simulink library "Springs_Axle3_Independent"  (R2026a)
settings: Solver=VariableStepAuto
libraries: fl_lib x6, Spring_Element x6
Description:
  | Component of Simscape Vehicle Templates Library
  | 
  | Copyright 2018-2026 The MathWorks, Inc.
settings Model: Creator=smiller  LastModifiedBy=smiller

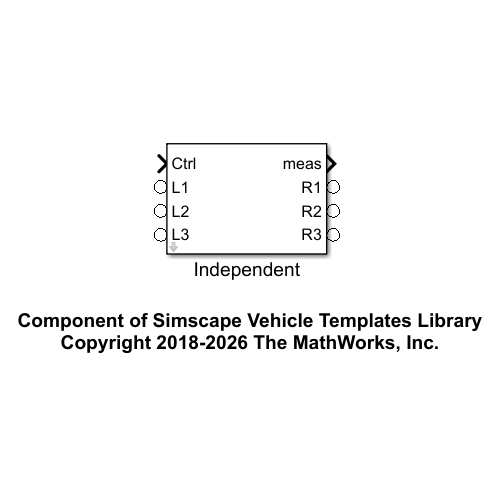
[thumbnail: Simulink's stored preview of the top-level diagram]
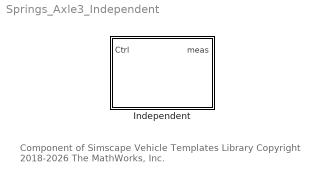
== system Springs_Axle3_Independent ==
  note: Component of Simscape Vehicle Templates Library
      | Copyright 2018-2026 The MathWorks, Inc.
  Independent : Subsystem  VariantControl=Independent  mask(Independent Springs){}
      mask help: Models independent left and right springs on three axles

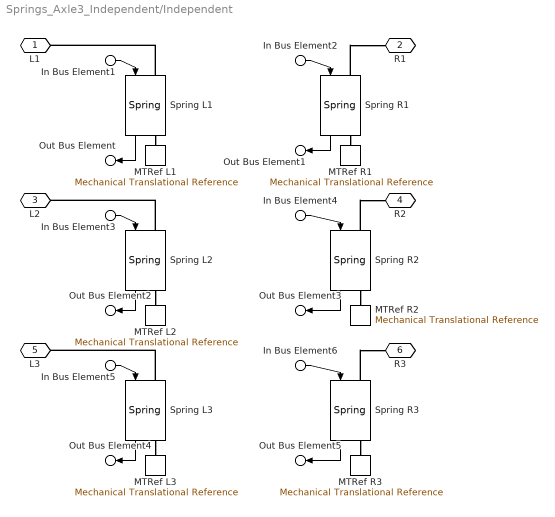
== system Springs_Axle3_Independent/Independent ==
  In Bus Element1 : Inport  PortName=Ctrl  Element=L1
  In Bus Element2 : Inport  PortName=Ctrl  Element=R1
  In Bus Element3 : Inport  PortName=Ctrl  Element=L2
  In Bus Element4 : Inport  PortName=Ctrl  Element=R2
  In Bus Element5 : Inport  PortName=Ctrl  Element=L3
  In Bus Element6 : Inport  PortName=Ctrl  Element=R3
  MTRef L1 : fl_lib/Mechanical/Translational Elements/Mechanical Translational Reference
  MTRef L2 : fl_lib/Mechanical/Translational Elements/Mechanical Translational Reference
  MTRef L3 : fl_lib/Mechanical/Translational Elements/Mechanical Translational Reference
  MTRef R1 : fl_lib/Mechanical/Translational Elements/Mechanical Translational Reference
  MTRef R2 : fl_lib/Mechanical/Translational Elements/Mechanical Translational Reference
  MTRef R3 : fl_lib/Mechanical/Translational Elements/Mechanical Translational Reference
  Spring L1 : Spring_Element/Spring  VariantControl=Variant1  LabelModeActiveChoice=Linear  Spring=Spring.Axle1  VariantLabel=Spring.Axle1.class.Value
      settings: AttributesFormatString=%<ActiveVariant>
  Spring L2 : Spring_Element/Spring  VariantControl=Variant1  LabelModeActiveChoice=Linear  Spring=Spring.Axle2  VariantLabel=Spring.Axle2.class.Value
      settings: AttributesFormatString=%<ActiveVariant>
  Spring L3 : Spring_Element/Spring  VariantControl=Variant1  LabelModeActiveChoice=Linear  Spring=Spring.Axle3  VariantLabel=Spring.Axle3.class.Value
      settings: AttributesFormatString=%<ActiveVariant>
  Spring R1 : Spring_Element/Spring  VariantControl=Variant1  LabelModeActiveChoice=Linear  Spring=Spring.Axle1  VariantLabel=Spring.Axle1.class.Value
      settings: AttributesFormatString=%<ActiveVariant>
  Spring R2 : Spring_Element/Spring  VariantControl=Variant1  LabelModeActiveChoice=Linear  Spring=Spring.Axle2  VariantLabel=Spring.Axle2.class.Value
      settings: AttributesFormatString=%<ActiveVariant>
  Spring R3 : Spring_Element/Spring  VariantControl=Variant1  LabelModeActiveChoice=Linear  Spring=Spring.Axle3  VariantLabel=Spring.Axle3.class.Value
      settings: AttributesFormatString=%<ActiveVariant>
  L1 : PMIOPort  Side=Left
  R1 : PMIOPort  Port=2  Side=Right
  L2 : PMIOPort  Port=3  Side=Left
  R2 : PMIOPort  Port=4  Side=Right
  L3 : PMIOPort  Port=5  Side=Left
  R3 : PMIOPort  Port=6  Side=Right
  Out Bus Element : Outport  VectorParamsAs1DForOutWhenUnconnected=off  PortName=meas  Element=L1
  Out Bus Element1 : Outport  VectorParamsAs1DForOutWhenUnconnected=off  PortName=meas  Element=R1
  Out Bus Element2 : Outport  VectorParamsAs1DForOutWhenUnconnected=off  PortName=meas  Element=L2
  Out Bus Element3 : Outport  VectorParamsAs1DForOutWhenUnconnected=off  PortName=meas  Element=R2
  Out Bus Element4 : Outport  VectorParamsAs1DForOutWhenUnconnected=off  PortName=meas  Element=L3
  Out Bus Element5 : Outport  VectorParamsAs1DForOutWhenUnconnected=off  PortName=meas  Element=R3
  wires:
  Spring R2/1 -> Out Bus Element3/1
  In Bus Element4/1 -> Spring R2/1
  Spring L2/1 -> Out Bus Element2/1
  In Bus Element3/1 -> Spring L2/1
  Spring R1/1 -> Out Bus Element1/1
  In Bus Element2/1 -> Spring R1/1
  Spring L1/1 -> Out Bus Element/1
  In Bus Element1/1 -> Spring L1/1
  In Bus Element5/1 -> Spring L3/1
  Spring L3/1 -> Out Bus Element4/1
  In Bus Element6/1 -> Spring R3/1
  Spring R3/1 -> Out Bus Element5/1
  connections:
  Spring L1/RConn1 -- MTRef L1/LConn1
  Spring L1/LConn1 -- L1/RConn1
  Spring L2/RConn1 -- MTRef L2/LConn1
  Spring L2/LConn1 -- L2/RConn1
  Spring R2/RConn1 -- MTRef R2/LConn1
  Spring R2/LConn1 -- R2/RConn1
  Spring R1/RConn1 -- MTRef R1/LConn1
  Spring R1/LConn1 -- R1/RConn1
  Spring R3/LConn1 -- R3/RConn1
  Spring R3/RConn1 -- MTRef R3/LConn1
  Spring L3/LConn1 -- L3/RConn1
  Spring L3/RConn1 -- MTRef L3/LConn1
